simulink model "HDLChannelEstimator"  (R2024a)
settings: Solver=FixedStepDiscrete  StartTime=0.0  StopTime=stopTime  RelTol=1e-3
undefined symbols (not defined in the file): CONST
libraries: HDL_ieee_8021513 x4, dspsrcs4 x3, whdlutilities x1, hdlsllib x1, whdlmod x1
settings Model: DataTypeOverride=Off  Creator=cotti  LastModifiedBy=cotti
settings OptimizationCC: BlockReduction=off  ConditionallyExecuteInputs=off  DefaultParameterBehavior=Inlined  InheritOutputTypeSmallerThanSingle=on
settings DebuggingCC: AlgebraicLoopMsg=error  ArtificialAlgebraicLoopMsg=error  SingleTaskRateTransMsg=error  UnconnectedInputMsg=warning  UnconnectedOutputMsg=warning  UnconnectedLineMsg=warning
settings HardwareCC: ProdBitPerPointer=32  ProdBitPerSizeT=32  ProdBitPerPtrDiffT=32  ProdLargestAtomicFloat=None  ProdIntDivRoundTo=Undefined  ProdEndianess=Unspecified  ProdWordSize=32  ProdHWDeviceType=ASIC/FPGA->ASIC/FPGA  TargetBitPerLong=64  TargetBitPerPointer=64  TargetBitPerSizeT=64  TargetBitPerPtrDiffT=64  TargetLongLongMode=on  TargetIntDivRoundTo=Zero  TargetEndianess=LittleEndian  TargetWordSize=64  TargetHWDeviceType=Custom Processor->MATLAB Host Computer  ProdEqTarget=off

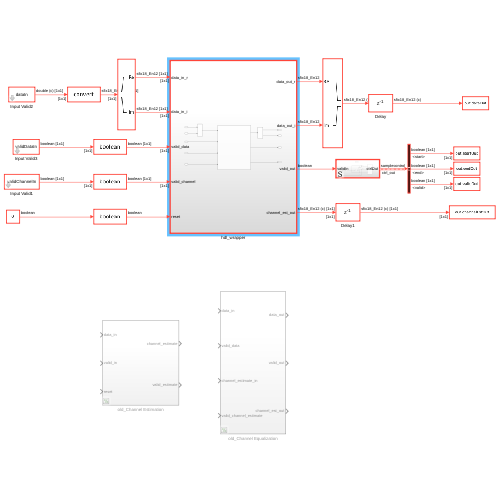
[thumbnail: Simulink's stored preview of the top-level diagram]
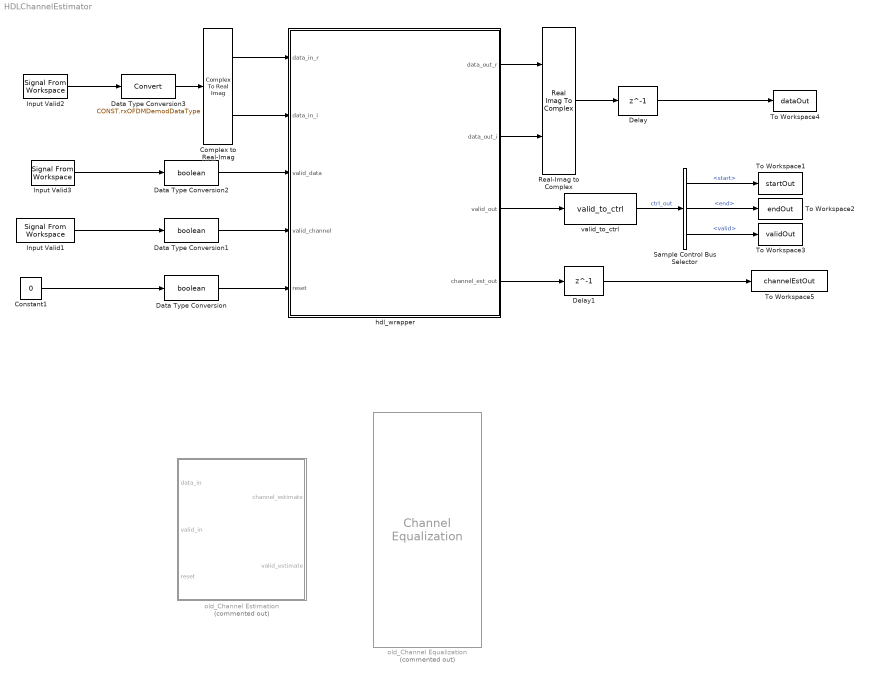
== system HDLChannelEstimator ==
  Complex to Real-Imag : ComplexToRealImag
  Constant1 : Constant  Value=0  OutDataTypeStr=boolean  SampleTime=-1
  Data Type Conversion : DataTypeConversion  OutDataTypeStr=boolean  SaturateOnIntegerOverflow=off  RndMeth=Floor
  Data Type Conversion1 : DataTypeConversion  OutDataTypeStr=boolean  SaturateOnIntegerOverflow=off  RndMeth=Floor
  Data Type Conversion2 : DataTypeConversion  OutDataTypeStr=boolean  SaturateOnIntegerOverflow=off  RndMeth=Floor
  Data Type Conversion3 : DataTypeConversion  OutDataTypeStr=CONST.rxOFDMDemodDataType  SaturateOnIntegerOverflow=off  RndMeth=Floor
  Delay : Delay  DelayLength=1  InitialCondition=0  UseCircularBuffer=on
  Delay1 : Delay  DelayLength=1  InitialCondition=0  UseCircularBuffer=on
  Input Valid1 : dspsrcs4/Signal From Workspace  X=validChannelIn  Ts=1/CONST.fPHY  nsamps=1  OutputAfterFinalValue=Setting to zero  ignoreOrWarnInputAndFrameLengths=off  OutputFrames=off
  Input Valid2 : dspsrcs4/Signal From Workspace  X=dataIn  Ts=1/CONST.fPHY  nsamps=1  OutputAfterFinalValue=Setting to zero  ignoreOrWarnInputAndFrameLengths=off  OutputFrames=off
  Input Valid3 : dspsrcs4/Signal From Workspace  X=validDataIn  Ts=1/CONST.fPHY  nsamps=1  OutputAfterFinalValue=Setting to zero  ignoreOrWarnInputAndFrameLengths=off  OutputFrames=off
  Real-Imag to Complex : RealImagToComplex
  Sample Control Bus Selector : whdlutilities/Sample Control Bus Selector  OutputSignals=start,end,valid
  To Workspace1 : ToWorkspace  VariableName=startOut  SampleTime=1/CONST.fPHY
      settings: Save2DSignal=2-D array (concatenate along first dimension)
  To Workspace2 : ToWorkspace  VariableName=endOut  SampleTime=1/CONST.fPHY
      settings: Save2DSignal=2-D array (concatenate along first dimension)
  To Workspace3 : ToWorkspace  VariableName=validOut  SampleTime=1/CONST.fPHY
      settings: Save2DSignal=2-D array (concatenate along first dimension)
  To Workspace4 : ToWorkspace  VariableName=dataOut  SampleTime=1/CONST.fPHY
      settings: Save2DSignal=2-D array (concatenate along first dimension)
  To Workspace5 : ToWorkspace  VariableName=channelEstOut  SampleTime=1/CONST.fPHY
      settings: Save2DSignal=2-D array (concatenate along first dimension)
  hdl_wrapper : Subsystem  TreatAsAtomicUnit=on
  old_Channel Equalization : HDL_ieee_8021513/channel_estimation_and_equalization/Channel Equalization  Commented=on  SystemSampleTime=-1  VariantActivationTime=update diagram  AllowFlexibleInterface=on  Latency=0  AutoFrameSizeCalculation=off
      settings: SourceProductName=HDL IEEE 8021513
  old_Channel Estimation : Subsystem  Commented=on
  valid_to_ctrl : HDL_ieee_8021513/valid_to_ctrl  SystemSampleTime=-1  VariantActivationTime=update diagram  AllowFlexibleInterface=on  Latency=0  AutoFrameSizeCalculation=off
      settings: SourceProductName=HDL IEEE 8021513
  wires:
  Constant1/1 -> Data Type Conversion/1
  Sample Control Bus Selector/2 -> To Workspace2/1  "<end>"
  Sample Control Bus Selector/1 -> To Workspace1/1  "<start>"
  Sample Control Bus Selector/3 -> To Workspace3/1  "<valid>"
  valid_to_ctrl/1 -> Sample Control Bus Selector/1  "ctrl_out"
  Delay/1 -> To Workspace4/1
  Delay1/1 -> To Workspace5/1
  Input Valid2/1 -> Data Type Conversion3/1
  Input Valid3/1 -> Data Type Conversion2/1
  Input Valid1/1 -> Data Type Conversion1/1
  Data Type Conversion2/1 -> hdl_wrapper/3(valid_data)
  Data Type Conversion1/1 -> hdl_wrapper/4(valid_channel)
  Data Type Conversion/1 -> hdl_wrapper/5(reset)
  hdl_wrapper/3(valid_out) -> valid_to_ctrl/1
  hdl_wrapper/4(channel_est_out) -> Delay1/1
  hdl_wrapper/1(data_out_r) -> Real-Imag to Complex/1
  hdl_wrapper/2(data_out_i) -> Real-Imag to Complex/2
  Real-Imag to Complex/1 -> Delay/1
  Data Type Conversion3/1 -> Complex to Real-Imag/1
  Complex to Real-Imag/1 -> hdl_wrapper/1(data_in_r)
  Complex to Real-Imag/2 -> hdl_wrapper/2(data_in_i)

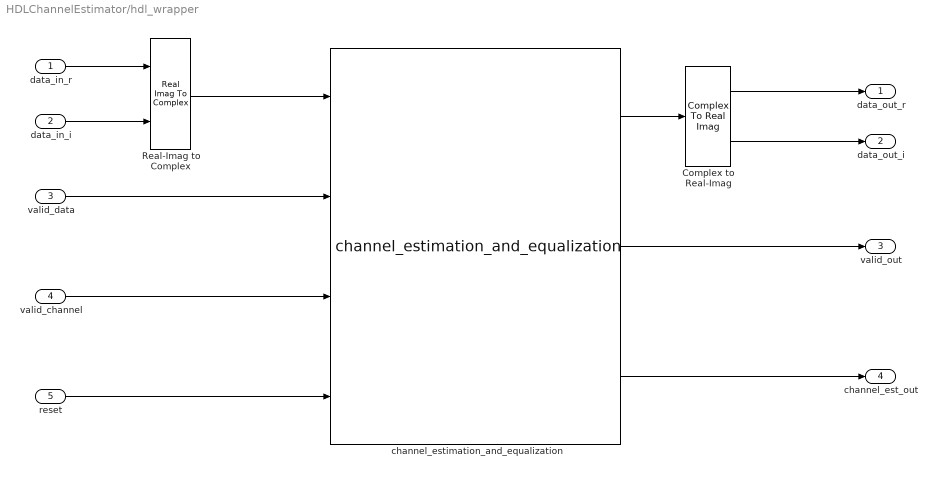
== system HDLChannelEstimator/hdl_wrapper ==
  data_in_r : Inport
  data_in_i : Inport  Port=2
  valid_data : Inport  Port=3
  valid_channel : Inport  Port=4
  reset : Inport  Port=5
  Complex to Real-Imag : ComplexToRealImag
  Real-Imag to Complex : RealImagToComplex
  channel_estimation_and_equalization : HDL_ieee_8021513/channel_estimation_and_equalization  SystemSampleTime=-1  VariantActivationTime=update diagram  AllowFlexibleInterface=on  Latency=0  AutoFrameSizeCalculation=off
      settings: SourceProductName=HDL IEEE 8021513
  data_out_r : Outport
  data_out_i : Outport  Port=2
  valid_out : Outport  Port=3
  channel_est_out : Outport  Port=4
  wires:
  valid_data/1 -> channel_estimation_and_equalization/2
  channel_estimation_and_equalization/3 -> channel_est_out/1
  channel_estimation_and_equalization/2 -> valid_out/1
  valid_channel/1 -> channel_estimation_and_equalization/3
  reset/1 -> channel_estimation_and_equalization/4
  data_in_r/1 -> Real-Imag to Complex/1
  data_in_i/1 -> Real-Imag to Complex/2
  Real-Imag to Complex/1 -> channel_estimation_and_equalization/1
  channel_estimation_and_equalization/1 -> Complex to Real-Imag/1
  Complex to Real-Imag/1 -> data_out_r/1
  Complex to Real-Imag/2 -> data_out_i/1

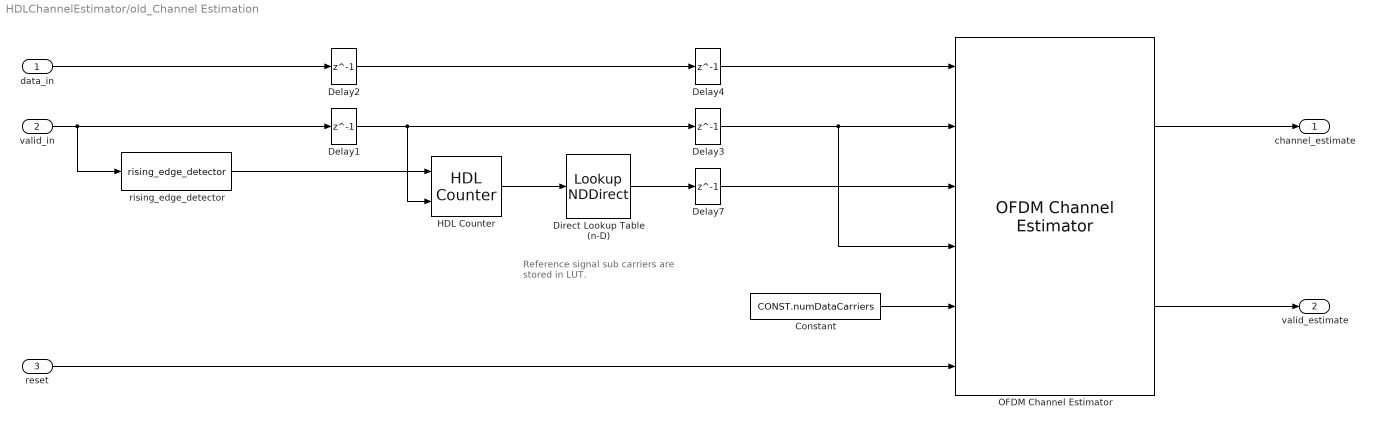
== system HDLChannelEstimator/old_Channel Estimation ==
  note: Reference signal sub carriers are stored in LUT.
  data_in : Inport
  valid_in : Inport  Port=2
  reset : Inport  Port=3
  Constant : Constant  Value=CONST.numDataCarriers  OutDataTypeStr=fixdt(0,nextpow2(CONST.numDataCarriers),0)  SampleTime=-1
  Delay{1..4,7} (5 alike) : Delay  DelayLength=1  InitialCondition=0
  Direct Lookup Table (n-D) : LookupNDDirect  NumberOfTableDimensions=1  Table=fi(CONST.channelEstReference, 1, CONST.rxChannelEstReferenceWordLength, CONST.rxChannelEstReferenceFractionLength)  DiagnosticForOutOfRangeInput=Error  RemoveProtectionInput=on  TableDataTypeStr=fixdt(1,16,12)
  HDL Counter : hdlsllib/Sources/HDL Counter  CountType=Count limited  CountInit=0  CountStep=1  CountMax=CONST.numDataCarriers-1  CountFromType=Initial value  CountFrom=0  CountResetPort=on  CountLoadPort=off  CountEnbPort=on  CountDirPort=off  CountHitOutputPort=off  CountDataType=Unsigned  CountWordLen=nextpow2(CONST.numDataCarriers)  CountFracLen=0  CountSampTime=1
  OFDM Channel Estimator : whdlmod/OFDM Channel Estimator  timeAvgCheckBox=on  numOFDMSymToBeAvg=2  enableInterpCheckBox=off  interpFac=3  maxNumSubCarPerSym=CONST.N  resetPort=on
  rising_edge_detector : HDL_ieee_8021513/rising_edge_detector  SystemSampleTime=-1  VariantActivationTime=update diagram  AllowFlexibleInterface=on  Latency=0  AutoFrameSizeCalculation=off
      settings: SourceProductName=HDL IEEE 8021513
  channel_estimate : Outport
  valid_estimate : Outport  Port=2
  wires:
  OFDM Channel Estimator/1 -> channel_estimate/1
  Constant/1 -> OFDM Channel Estimator/5
  valid_in/1 -> rising_edge_detector/1, Delay1/1
  Direct Lookup Table (n-D)/1 -> Delay7/1
  OFDM Channel Estimator/2 -> valid_estimate/1
  data_in/1 -> Delay2/1
  Delay1/1 -> HDL Counter/2, Delay3/1
  HDL Counter/1 -> Direct Lookup Table (n-D)/1
  Delay4/1 -> OFDM Channel Estimator/1
  Delay7/1 -> OFDM Channel Estimator/3
  Delay3/1 -> OFDM Channel Estimator/4, OFDM Channel Estimator/2
  Delay2/1 -> Delay4/1
  rising_edge_detector/1 -> HDL Counter/1
  reset/1 -> OFDM Channel Estimator/6
